simulink model "QuarterCar_Validation"  (R2026a)
settings: Solver=ode45  StopTime=7  MaxStep=0.001  RelTol=1e-6
undefined symbols (not defined in the file): cs, ks, kt, ms, mu
settings Model: Creator=maitr  LastModifiedBy=maitr

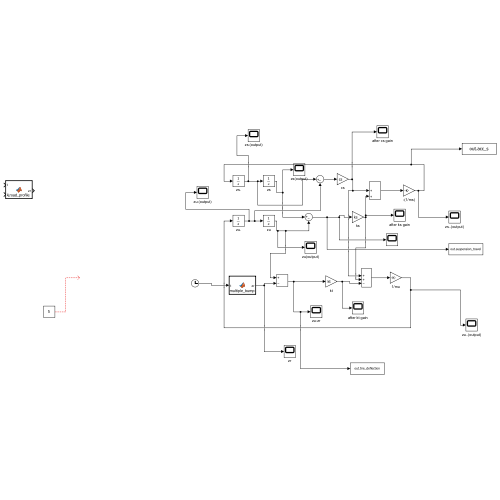
[thumbnail: Simulink's stored preview of the top-level diagram]
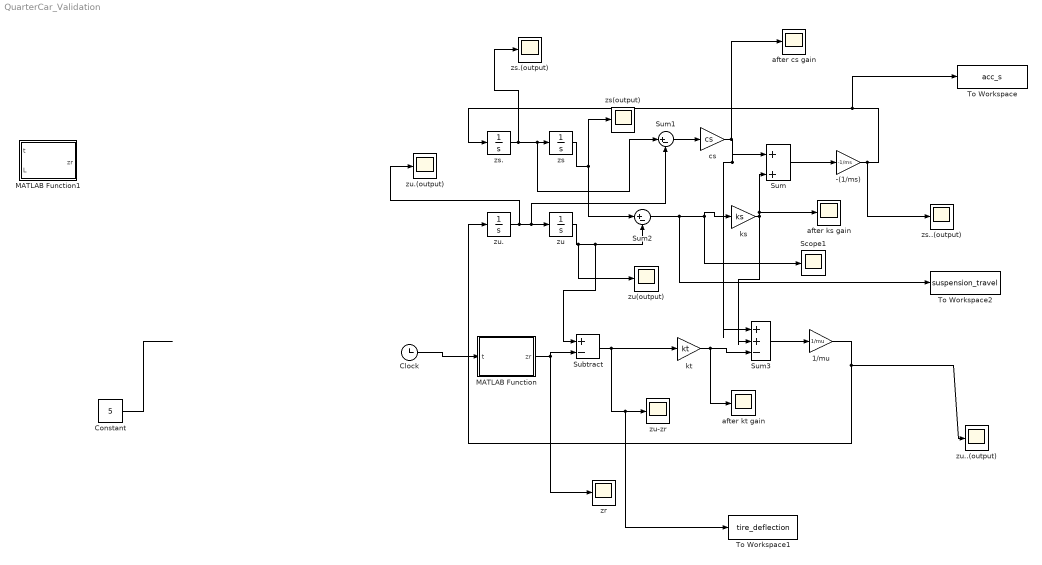
== system QuarterCar_Validation ==
  -(1/ms) : Gain  Gain=-1/ms
  1/mu : Gain  Gain=1/mu
  Clock : Clock
  Constant : Constant  Value=5
  MATLAB Function : MATLAB Function  TreatAsAtomicUnit=on
  MATLAB Function1 : MATLAB Function  TreatAsAtomicUnit=on
  Scope1 : Scope
      settings: DataLoggingVariableName=ScopeData5
  Subtract : Sum  Inputs=+-
  Sum : Sum  Inputs=|++
  Sum1 : Sum  Inputs=|+-
  Sum2 : Sum  Inputs=|+-
  Sum3 : Sum  Inputs=|++-
  To Workspace : ToWorkspace  VariableName=acc_s  SampleTime=-1
  To Workspace1 : ToWorkspace  VariableName=tire_deflection  SaveFormat=Timeseries  SampleTime=-1
  To Workspace2 : ToWorkspace  VariableName=suspension_travel  SaveFormat=Timeseries  SampleTime=-1
  after cs gain : Scope
      settings: ActiveDisplayYMinimum=-1  ActiveDisplayYMaximum=1  DataLoggingVariableName=ScopeData7
  after ks gain : Scope
      settings: ActiveDisplayYMinimum=-1  ActiveDisplayYMaximum=1  DataLoggingVariableName=ScopeData8
  after kt gain : Scope
      settings: ActiveDisplayYMinimum=-1  ActiveDisplayYMaximum=1  DataLoggingVariableName=ScopeData9
  cs : Gain  Gain=cs
  ks : Gain  Gain=ks
  kt : Gain  Gain=kt
  zr : Scope
      settings: ActiveDisplayYMinimum=-0.012499999999999997  ActiveDisplayYMaximum=0.1125
  zs : Integrator
  zs(output) : Scope
      settings: ActiveDisplayYMinimum=-0.051575890546753059  ActiveDisplayYMaximum=0.087060863952305459
  zs. : Integrator
  zs.(output) : Scope
      settings: ActiveDisplayYMinimum=-0.087337250817641154  ActiveDisplayYMaximum=0.07560187640950182  DataLoggingVariableName=ScopeData10
  zs..(output) : Scope
      settings: ActiveDisplayYMinimum=-9.25853049874584  ActiveDisplayYMaximum=9.9748311143069923  DataLoggingVariableName=ScopeData3
  zu : Integrator
  zu(output) : Scope
      settings: ActiveDisplayYMinimum=-0.018358738313139958  ActiveDisplayYMaximum=0.12310617090532706  DataLoggingVariableName=ScopeData2
  zu-zr : Scope
      settings: ActiveDisplayYMinimum=-1  ActiveDisplayYMaximum=1  DataLoggingVariableName=ScopeData6
  zu. : Integrator
  zu.(output) : Scope
      settings: ActiveDisplayYMinimum=-0.11204319110747693  ActiveDisplayYMaximum=0.093968203567396047  DataLoggingVariableName=ScopeData11
  zu..(output) : Scope
      settings: ActiveDisplayYMinimum=-1  ActiveDisplayYMaximum=1  DataLoggingVariableName=ScopeData4
  wires:
  zs./1 -> zs.(output)/1, Sum1/1, zs/1
  zu./1 -> zu.(output)/1, Sum1/2, zu/1
  Sum1/1 -> cs/1
  zs/1 -> zs(output)/1, Sum2/1
  zu/1 -> zu(output)/1, Sum2/2, Subtract/1
  Sum2/1 -> To Workspace2/1, ks/1, Scope1/1
  cs/1 -> after cs gain/1, Sum3/1, Sum/1
  ks/1 -> after ks gain/1, Sum/2, Sum3/2
  Sum/1 -> -(1/ms)/1
  -(1/ms)/1 -> zs..(output)/1, To Workspace/1, zs./1
  kt/1 -> after kt gain/1, Sum3/3
  Sum3/1 -> 1/mu/1
  1/mu/1 -> zu./1, zu..(output)/1
  MATLAB Function/1(zr) -> Subtract/2, zr/1
  Clock/1 -> MATLAB Function/1(t)
  Constant/1 -> ?
  Subtract/1 -> To Workspace1/1, zu-zr/1, kt/1

== matlab function QuarterCar_Validation/MATLAB Function ==
  data: t input; zr output
function zr = multiple_bump(t)

% Multiple-bump road profile
% Based on the validation case in the reference paper

zr = 0;

if t >= 0.5 && t <= 0.75

    a = 0.10;
    zr = a/2 * (1 - cos(8*pi*t));

elseif t >= 3.0 && t <= 3.25

    a = 0.05;
    zr = a/2 * (1 - cos(8*pi*t));

elseif t >= 5.0 && t <= 5.25

    a = 0.10;
    zr = a/2 * (1 - cos(8*pi*t));

else

    zr = 0;

end

== matlab function QuarterCar_Validation/MATLAB Function1 ==
  data: t input; zr output; L input
function zr = Lroad_profile(t,L)

h = 0.1;        % bump height (m)
v = 40/3.6;     % vehicle velocity (m/s)
d = 0;          % approach distance (m)

if t < d/v
    zr = 0;

elseif t <= (d+L)/v
    zr = h*sin((pi/L)*(v*t-d));

else
    zr = 0;
end
